simulink model "Cowley_315Exam2TakeHomeSim"  (R2020b)
settings: Solver=FixedStepAuto  StartTime=0.0  StopTime=2  FixedStep=0.001  RelTol=1e-3
values from neighbouring files (symbols this model uses):
  f0 = F/m    (= 20)    [Cowley_315Exam2TakeHome.m]    (also in Cowley_315Week8HW_Prob2.m = 2.5; ForceInputResponse.m = 2.5; VibeTribe_315GroupProjectSim.m = 7.3575)
  k = 1    [Cowley_315Exam2TakeHome.m]    (also in Cowley_315Week4HW_Problem3.m = 100; Cowley_315Week8HW_Prob1.m = 400000; Cowley_315Week8HW_Prob2.m = 500; Cowley_FinalTakeHome1.m = [k1 k2])
  m = 1    [Cowley_315Exam2TakeHome.m]    (also in Cowley_315Week4HW_Problem3.m = 10; Cowley_315Week8HW_Prob1.m = 1007; Cowley_315Week8HW_Prob2.m = 0.4; Cowley_FinalTakeHome1.m = [m1 m2])
  v0 = 0    [Cowley_315Exam2TakeHome.m]    (also in Cowley_315Week13HW_Problem1.m = [0;0]; Cowley_315Week13HW_Problem2.m = [0;0;1]; Cowley_315Week13_Problem3.m = [1 0]; Cowley_315Week4HW_Problem3.m = 10)
  w = 30    [Cowley_315Exam2TakeHome.m]    (also in Cowley_315Week8HW_Prob2.m = 10; Cowley_FinalTakeHome1.m = 1; Cowley_FinalTakeHome234.m = 2; Cowley_FinalTakeHome5.m = 0)
  x0 = 0    [Cowley_315Exam2TakeHome.m]    (also in Cowley_315Week13HW_Problem1.m = [0.1;1]; Cowley_315Week13HW_Problem2.m = zeros(3,1); Cowley_315Week13_Problem3.m = [0 0.1]; Cowley_315Week4HW_Problem3.m)
settings Model: Creator=mattcowley  LastModifiedBy=mattcowley

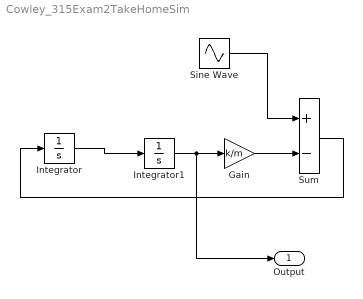
== system Cowley_315Exam2TakeHomeSim ==
  Gain : Gain  Gain=k/m
  Integrator : Integrator  InitialCondition=v0
  Integrator1 : Integrator  InitialCondition=x0
  Sine Wave : Sin  Amplitude=f0  Frequency=w  Phase=pi/2  SampleTime=0
  Sum : Sum  Inputs=+-
  Output : Outport  SignalName=x
  wires:
  Integrator/1 -> Integrator1/1
  Integrator1/1 -> Output/1, Gain/1
  Gain/1 -> Sum/2
  Sine Wave/1 -> Sum/1
  Sum/1 -> Integrator/1
